simulink model "Spring_Mass_Damper_Simulation"  (R2024a)
settings: Solver=VariableStepAuto  StartTime=0.0  StopTime=10.0  RelTol=1e-3
libraries: simulink x1
settings Model: Creator=HP  LastModifiedBy=HP

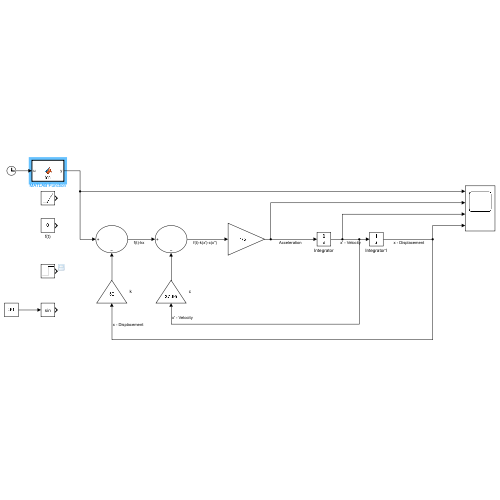
[thumbnail: Simulink's stored preview of the top-level diagram]
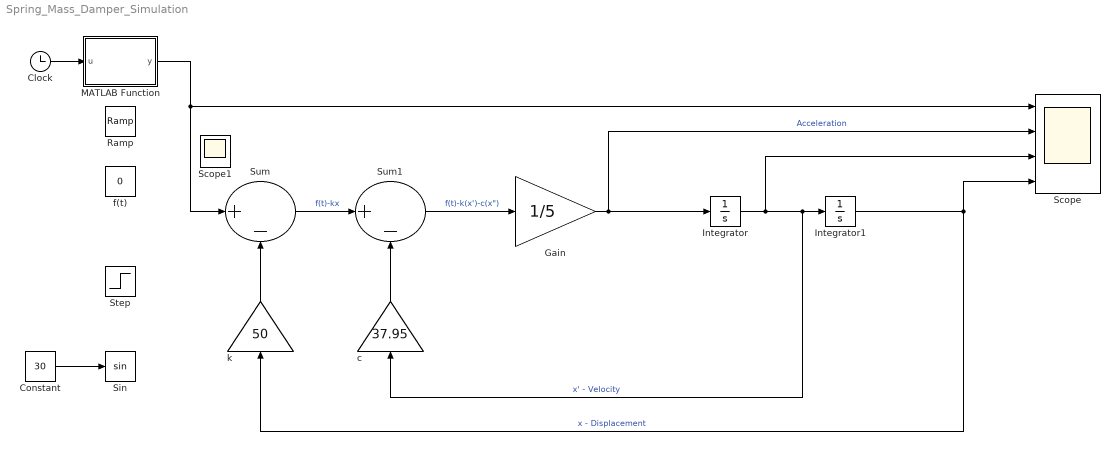
== system Spring_Mass_Damper_Simulation ==
  Clock : Clock
  Constant : Constant  Value=30
  Gain : Gain  Gain=1/5
  Integrator : Integrator
  Integrator1 : Integrator  InitialCondition=0.01
  MATLAB Function : MATLAB Function  TreatAsAtomicUnit=on
  Ramp : simulink/Sources/Ramp  slope=2  start=0  InitialOutput=0
  Scope : Scope  NumInputPorts=4
  Sin : Trigonometry
  Step : Step  After=5  SampleTime=0
  Sum : Sum  Inputs=|+-
  Sum1 : Sum  Inputs=|+-
  c : Gain  Gain=37.95
  f(t) : Constant  Value=0
  k : Gain  Gain=50
  Scope1 : Scope
  wires:
  k/1 -> Sum/2
  Integrator1/1 -> k/1, Scope/4  "x - Displacement"
  Integrator/1 -> Scope/3, c/1, Integrator1/1  "x' - Velocity"
  Sum/1 -> Sum1/1  "f(t)-kx"
  c/1 -> Sum1/2
  Sum1/1 -> Gain/1  "f(t)-k(x')-c(x\")"
  Gain/1 -> Scope/2, Integrator/1  "Acceleration"
  Constant/1 -> Sin/1
  Clock/1 -> MATLAB Function/1(u)
  MATLAB Function/1(y) -> Scope/1, Sum/1

== matlab function Spring_Mass_Damper_Simulation/MATLAB Function ==
  data: u input; y output
function y = fcn(u)
f=1.0;
a=1;
w=2*pi*f;
y = a*sin(w*u);
